simulink model "precom_dyn_1"  (R2018b)
settings: Solver=FixedStepAuto  StartTime=0.0  StopTime=5  FixedStep=.001  RelTol=1e-3  EnableMultiTasking=on
undefined symbols (not defined in the file): A, B, C, F1, K1, precomp_stat
libraries: cstblocks x5, simulink x1
settings Model: Creator=user  LastModifiedBy=牟城志
settings SolverCC: ZeroCrossControl=EnableAll  PositivePriorityOrder=on
settings DataIOCC: SaveFormat=Array  SignalLoggingSaveFormat=ModelDataLogs
settings OptimizationCC: BooleanDataType=off  InitFltsAndDblsToZero=on  LifeSpan=inf
settings DebuggingCC: SaveWithParameterizedLinksMsg=none  UnderspecifiedInitializationDetection=Classic  MergeDetectMultiDrivingBlocksExec=none  SignalResolutionControl=TryResolveAllWithWarning  MultiTaskDSMMsg=warning  MultiTaskCondExecSysMsg=none  FcnCallInpInsideContextMsg=warning  SFUnexpectedBacktrackingDiag=warning  SFNoUnconditionalDefaultTransitionDiag=warning  SFExecutionAtInitializationDiag=none
settings HardwareCC: ProdBitPerPointer=32  ProdBitPerSizeT=32  ProdBitPerPtrDiffT=32  ProdLargestAtomicFloat=None  ProdIntDivRoundTo=Undefined  ProdEndianess=Unspecified  ProdWordSize=32  ProdHWDeviceType=32-bit Generic  TargetUnknown=on
settings ModelReferenceCC: PropagateSignalLabelsOutOfModel=off
settings SFSimCC: SimUseLocalCustomCode=off
settings RTWCC: RTWUseLocalCustomCode=off
settings CodeAppCC: StateflowObjectComments=on
settings GRTTargetCC: TargetFcnLib=ansi_tfl_tmw.mat  TargetLangStandard=C89/C90 (ANSI)  GeneratePreprocessorConditionals=Disable all  CombineOutputUpdateFcns=off  GRTInterface=on
settings ConfigComp: CovMetricSettings=dw  CovHtmlReporting=on  CovSaveCumulativeToWorkspaceVar=on  CovSaveSingleToWorkspaceVar=on  CovExternalEMLEnable=off

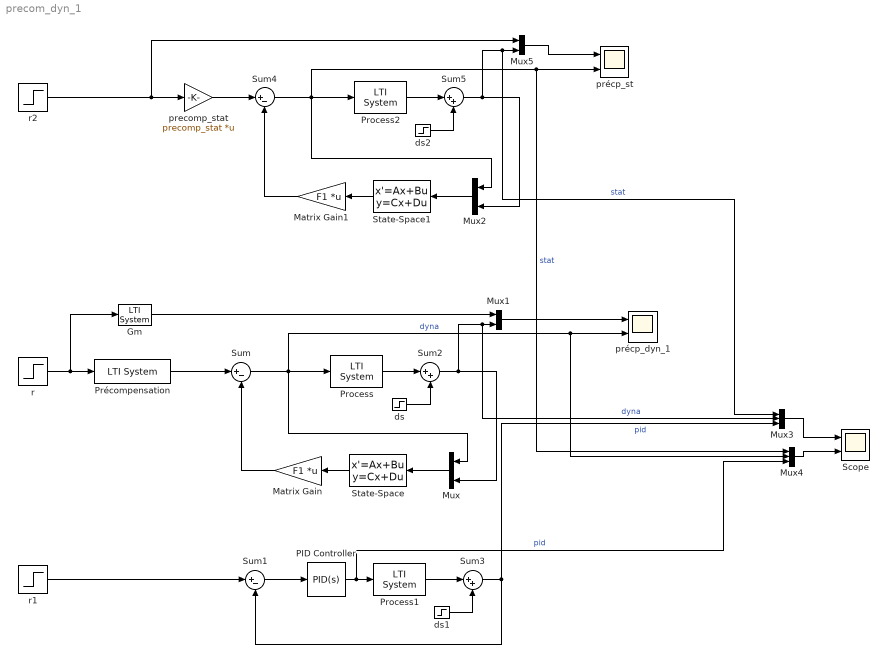
== system precom_dyn_1 ==
  Gm : cstblocks/LTI System  sys=Gm1  IC=[]
  Matrix Gain : Gain  Gain=F1  Multiplication=Matrix(K*u)  SaturateOnIntegerOverflow=on  OutDataTypeStr=Inherit: Same as input  ParamDataTypeStr=Inherit: Same as input
  Matrix Gain1 : Gain  Gain=F1  Multiplication=Matrix(K*u)  SaturateOnIntegerOverflow=on  OutDataTypeStr=Inherit: Same as input  ParamDataTypeStr=Inherit: Same as input
  Mux{,1..2,5} (4 alike) : Mux  Inputs=2
  Mux3 : Mux  Inputs=3
  Mux4 : Mux  Inputs=3
  PID Controller : simulink/Continuous/PID Controller  Controller=PID  Form=Parallel  TimeDomain=Continuous-time  SampleTime=-1  IntegratorMethod=Forward Euler  FilterMethod=Forward Euler  ControllerParametersSource=internal  P=0.228829303316168  I=0.317666235926833  D=0.0395981827262747  UseFilter=on  N=270.054568931008  TunerSelectOption=Transfer Function Based (PID Tuner App)  InitialConditionSource=internal  InitialConditionForIntegrator=0  InitialConditionForFilter=0  DifferentiatorICPrevScaledInput=0  ExternalReset=none  TrackingMode=off  Kt=1  LimitOutput=on  UpperSaturationLimit=6  LowerSaturationLimit=-6  LinearizeAsGain=on  AntiWindupMode=none  Kb=1  POutMin=[]  POutMax=[]  IOutMin=[]  IOutMax=[]  DOutMin=[]  DOutMax=[]  NOutMin=[]  NOutMax=[]  SumOutMin=[]  SumOutMax=[]  SaturationOutMin=[]  SaturationOutMax=[]  PParamMin=[]  PParamMax=[]  IParamMin=[]  IParamMax=[]  DParamMin=[]  DParamMax=[]  NParamMin=[]  NParamMax=[]  KbParamMin=[]  KbParamMax=[]  KtParamMin=[]  KtParamMax=[]  KbOutMin=[]  KbOutMax=[]  KtOutMin=[]  KtOutMax=[]  IntegratorOutMin=[]  IntegratorOutMax=[]  FilterOutMin=[]  FilterOutMax=[]  SumI1OutMin=[]  SumI1OutMax=[]  SumI2OutMin=[]  SumI2OutMax=[]  SumI3OutMin=[]  SumI3OutMax=[]  SumI4OutMin=[]  SumI4OutMax=[]  SumDOutMin=[]  SumDOutMax=[]  DifferentiatorOutMin=[]  DifferentiatorOutMax=[]  FilterDiffOutCoefMin=[]  FilterDiffOutCoefMax=[]  ReciprocalOutMin=[]  ReciprocalOutMax=[]  SumDenOutMin=[]  SumDenOutMax=[]  SumNumOutMin=[]  SumNumOutMax=[]  DivideOutMin=[]  DivideOutMax=[]  IntegratorContinuousStateAttributes=''  IntegratorStateMustResolveToSignalObject=off  IntegratorRTWStateStorageClass=Auto  FilterContinuousStateAttributes=''  FilterStateMustResolveToSignalObject=off  FilterRTWStateStorageClass=Auto  ParallelPVariant=InternalParameters  IdealPVariant=Disabled  IVariant=InternalParameters  DVariant=InternalParameters  IntegratorVariant=Continuous  SatVariant=Enabled  AWVariant=Passthrough  PCopyVariant=Disabled  TRVariant=Disabled  FdbkBlocksVariant=Forward  IdealPFdbkVariant=Disabled  SatFdbkVariant=Disabled  DerivativeFilterVariant=ContFilter  NVariant=InternalParameters  NCopyVariant=Disabled  FilterICVariant=InternalICsFilter  IntegratorICVariant=InternalICs  ExternalResetVariant=Disabled  TRSumVariant=Passthrough  SumFdbkVariant=Disabled  SumVariant=Sum_PID
  Process : cstblocks/LTI System  sys=G  IC=[]
  Process1 : cstblocks/LTI System  sys=G  IC=[]
  Process2 : cstblocks/LTI System  sys=G  IC=[]
  Précompensation : cstblocks/LTI System  sys=Precomp  IC=[]
  Scope : Scope  NumInputPorts=2
  State-Space : StateSpace  A=A-K1*C  B=[B K1]  C=eye(3)  D=[0 0 ;0 0 ;0 0 ]  InitialCondition=0
  State-Space1 : StateSpace  A=A-K1*C  B=[B K1]  C=eye(3)  D=[0 0 ;0 0 ;0 0 ]  InitialCondition=0
  Sum : Sum  Inputs=|+-  SaturateOnIntegerOverflow=on  InputSameDT=on  OutDataTypeStr=Inherit: Same as first input
  Sum1 : Sum  Inputs=|+-  SaturateOnIntegerOverflow=on  InputSameDT=on  OutDataTypeStr=Inherit: Same as first input
  Sum2 : Sum  Inputs=|++  SaturateOnIntegerOverflow=on  InputSameDT=on  OutDataTypeStr=Inherit: Same as first input
  Sum3 : Sum  Inputs=|++  SaturateOnIntegerOverflow=on  InputSameDT=on  OutDataTypeStr=Inherit: Same as first input
  Sum4 : Sum  Inputs=|+-  SaturateOnIntegerOverflow=on  InputSameDT=on  OutDataTypeStr=Inherit: Same as first input
  Sum5 : Sum  Inputs=|++  SaturateOnIntegerOverflow=on  InputSameDT=on  OutDataTypeStr=Inherit: Same as first input
  ds : Step  Time=3  SampleTime=0
  ds1 : Step  Time=3  SampleTime=0
  ds2 : Step  Time=3  SampleTime=0
  precomp_stat : Gain  Gain=precomp_stat  Multiplication=Matrix(K*u)  SaturateOnIntegerOverflow=on  OutDataTypeStr=Inherit: Same as input  ParamDataTypeStr=Inherit: Same as input
  précp_dyn_1 : Scope  NumInputPorts=2
  précp_st : Scope  NumInputPorts=2
  r : Step  SampleTime=0
  r1 : Step  SampleTime=0
  r2 : Step  SampleTime=0
  wires:
  r/1 -> Précompensation/1, Gm/1
  Process/1 -> Sum2/1
  Mux1/1 -> précp_dyn_1/1
  Sum2/1 -> Mux/2, Mux3/2, Mux1/2  "dyna"
  Sum/1 -> Mux4/2, précp_dyn_1/2, Process/1, Mux/1  "dyna"
  Matrix Gain/1 -> Sum/2
  State-Space/1 -> Matrix Gain/1
  Mux/1 -> State-Space/1
  Gm/1 -> Mux1/1
  Précompensation/1 -> Sum/1
  ds/1 -> Sum2/2
  r1/1 -> Sum1/1
  Sum1/1 -> PID Controller/1
  PID Controller/1 -> Mux4/3, Process1/1  "pid"
  ds1/1 -> Sum3/2
  Process1/1 -> Sum3/1
  Mux3/1 -> Scope/1
  Mux4/1 -> Scope/2
  ds2/1 -> Sum5/2
  Process2/1 -> Sum5/1
  r2/1 -> precomp_stat/1, Mux5/1
  Sum5/1 -> Mux2/2, Mux3/1, Mux5/2  "stat"
  Mux2/1 -> State-Space1/1
  Sum4/1 -> Mux4/1, précp_st/2, Process2/1, Mux2/1  "stat"
  State-Space1/1 -> Matrix Gain1/1
  Matrix Gain1/1 -> Sum4/2
  precomp_stat/1 -> Sum4/1
  Mux5/1 -> précp_st/1
  Sum3/1 -> Mux3/3, Sum1/2  "pid"
